simulink model "forcaster"  (Simulink 10.1)
settings: Solver=FixedStepAuto  StartTime=0.0  StopTime=10.0  FixedStep=DT  RelTol=1e-3
values from neighbouring files (symbols this model uses):
  T_s = 0.1    [run_Top_Model.m]
undefined symbols (not defined in the file or in its folder): DiscIntNeverNeededParam, T_mean, T_r
libraries: ctrlSharedLib x2, dspmtrx3 x1
settings Model: Creator=lpwoolcock  LastModifiedBy=arthu
settings DataIOCC: SaveFormat=Dataset  ReturnWorkspaceOutputs=on
settings OptimizationCC: LifeSpan=auto
settings DebuggingCC: UnderspecifiedInitializationDetection=Simplified  MergeDetectMultiDrivingBlocksExec=error  SFUnexpectedBacktrackingDiag=error  SFNoUnconditionalDefaultTransitionDiag=error  SFExecutionAtInitializationDiag=warning  ArithmeticOperatorsInVariantConditions=error
settings HardwareCC: ProdBitPerPointer=64  ProdBitPerSizeT=64  ProdBitPerPtrDiffT=64  ProdLargestAtomicFloat=Float  ProdIntDivRoundTo=Zero  ProdEndianess=LittleEndian  ProdWordSize=64  ProdHWDeviceType=Intel->x86-64 (Windows64)
settings ModelReferenceCC: PropagateSignalLabelsOutOfModel=on
settings SFSimCC: SimUseLocalCustomCode=on  CustomCodeUndefinedFunction=FilterOut
settings RTWCC: RTWUseLocalCustomCode=on
settings CodeAppCC: StateflowObjectComments=off
settings GRTTargetCC: TargetLangStandard=C99 (ISO)  CombineOutputUpdateFcns=on  GRTInterface=off
settings ConfigComp: CovMetricSettings=dwe  CovHtmlReporting=off  CovSaveCumulativeToWorkspaceVar=off  CovSaveSingleToWorkspaceVar=off  CovExternalEMLEnable=on

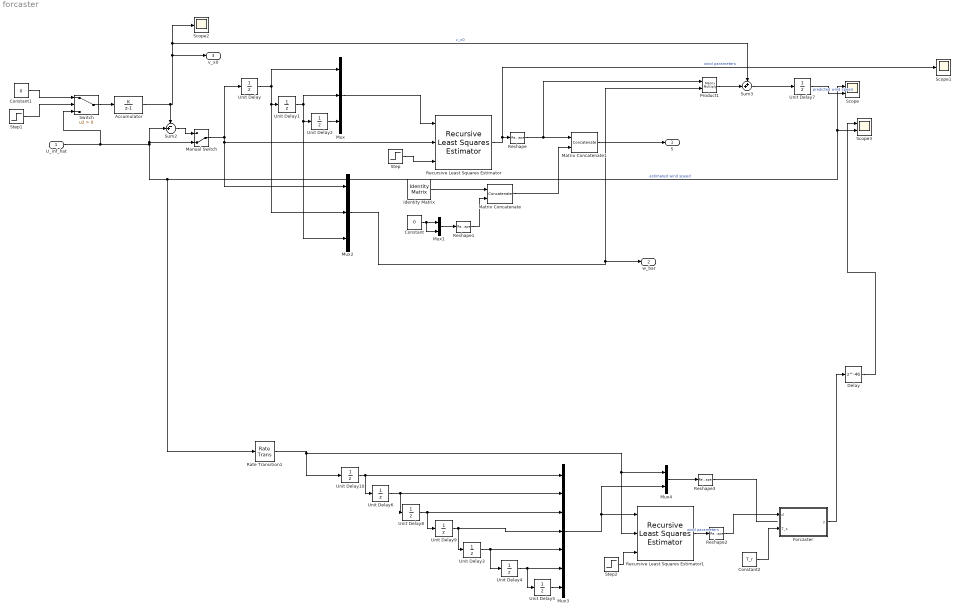
== system forcaster ==
  U_inf_hat : Inport  SampleTime=T_s
  Accumulator : DiscreteIntegrator  IntegratorMethod=Accumulation: Forward Euler  gainval=T_s/T_mean  SampleTime=T_s  ICPrevOutput=DiscIntNeverNeededParam  ICPrevScaledInput=DiscIntNeverNeededParam
  Constant : Constant  Value=0
  Constant1 : Constant  Value=0
  Constant2 : Constant  Value=T_r
  Delay : Delay  DelayLength=46  InitialCondition=0
  Forcaster : MATLAB Function  TreatAsAtomicUnit=on
  Identity Matrix : dspmtrx3/Identity Matrix  Inherit=off  N=2  Ts=T_s  dataType=double  isSigned=on  wordLen=16  udDataType=sfix(16)  fracBitsMode=Best precision  numFracBits=15  OutDataTypeStr=double  LastOutDataTypeStr=double
  Manual Switch : ManualSwitch  CurrentSetting=0
  Matrix Concatenate : Concatenate  Mode=Multidimensional array  ConcatenateDimension=2
  Matrix Concatenate1 : Concatenate  Mode=Multidimensional array
  Mux : Mux  Inputs=3
  Mux1 : Mux  Inputs=2
  Mux2 : Mux  Inputs=3
  Mux3 : Mux  Inputs=7
  Mux4 : Mux  Inputs=2
  Product1 : Product  Multiplication=Matrix(*)
  Rate Transition1 : RateTransition  Deterministic=off  OutPortSampleTime=T_r
  Recursive Least Squares Estimator : ctrlSharedLib/Recursive Least Squares Estimator  InitialEstimateSource=None  InitialParameterData=3  P0=1e4  InitialRegressors=0  InitialOutputs=0  History=Infinite  WindowLength=200  EstimationMethod=Forgetting Factor  AdaptationParameter=0.9  HasTimeVaryingAdaptationParameter=off  NormalizationBias=eps  OutputError=off  OutputP=off  AddEnablePort=off  ExternalReset=Rising  InputProcessing=Sample-based  Ts=-1
      settings: SourceProductBaseCode=CT,ID
  Recursive Least Squares Estimator1 : ctrlSharedLib/Recursive Least Squares Estimator  InitialEstimateSource=None  InitialParameterData=7  P0=1e4  InitialRegressors=0  InitialOutputs=0  History=Infinite  WindowLength=200  EstimationMethod=Forgetting Factor  AdaptationParameter=0.99  HasTimeVaryingAdaptationParameter=off  NormalizationBias=eps  OutputError=off  OutputP=off  AddEnablePort=off  ExternalReset=Rising  InputProcessing=Sample-based  Ts=T_r
      settings: SourceProductBaseCode=CT,ID
  Reshape : Reshape  OutputDimensionality=Row vector (2-D)
  Reshape1 : Reshape  OutputDimensionality=Column vector (2-D)
  Reshape2 : Reshape  OutputDimensionality=Row vector (2-D)
  Reshape3 : Reshape  OutputDimensionality=Column vector (2-D)
  Scope : Scope  NumInputPorts=2
  Scope1 : Scope
  Scope2 : Scope
  Scope3 : Scope  NumInputPorts=2
  Step : Step  Time=T_mean  SampleTime=T_s
  Step1 : Step  Time=T_mean  SampleTime=T_s
  Step2 : Step  Time=T_mean  SampleTime=T_s
  Sum2 : Sum  Inputs=-+|
  Sum3 : Sum  Inputs=++|
  Switch : Switch  Criteria=u2 > Threshold
  Unit Delay{,1..10} (11 alike) : UnitDelay  SampleTime=-1  HasFrameUpgradeWarning=on
  S : Outport  SampleTime=T_s
  w_bar : Outport  Port=2  SampleTime=T_s
  v_x0 : Outport  Port=3  SampleTime=T_s
  wires:
  Matrix Concatenate/1 -> Matrix Concatenate1/2
  Mux/1 -> Recursive Least Squares Estimator/1
  Unit Delay2/1 -> Mux/3
  Matrix Concatenate1/1 -> S/1
  Reshape/1 -> Product1/1, Matrix Concatenate1/1
  Constant/1 -> Mux1/2, Mux1/1
  Reshape1/1 -> Matrix Concatenate/2
  Mux1/1 -> Reshape1/1
  Unit Delay1/1 -> Mux/2, Mux2/3, Unit Delay2/1
  Recursive Least Squares Estimator/1 -> Scope1/1, Reshape/1  "wind parameters"
  Identity Matrix/1 -> Matrix Concatenate/1
  Unit Delay/1 -> Mux/1, Mux2/2, Unit Delay1/1
  Mux2/1 -> w_bar/1, Product1/2
  Unit Delay7/1 -> Scope/2  "predicted wind speed"
  U_inf_hat/1 -> Switch/3, Manual Switch/2, Sum2/2, Rate Transition1/1, Scope/1, Scope3/2  "estimated wind speed"
  Manual Switch/1 -> Mux2/1, Recursive Least Squares Estimator/2, Unit Delay/1
  Sum3/1 -> Unit Delay7/1
  Step/1 -> Recursive Least Squares Estimator/3
  Step1/1 -> Switch/2
  Constant1/1 -> Switch/1
  Switch/1 -> Accumulator/1
  Accumulator/1 -> Sum2/1, v_x0/1, Sum3/1, Scope2/1  "v_x0"
  Product1/1 -> Sum3/2
  Constant2/1 -> Forcaster/2(T_s)
  Sum2/1 -> Manual Switch/1
  Unit Delay5/1 -> Mux3/7
  Unit Delay4/1 -> Unit Delay5/1, Mux3/6
  Unit Delay3/1 -> Unit Delay4/1, Mux3/5
  Unit Delay9/1 -> Unit Delay3/1, Mux3/4
  Unit Delay8/1 -> Unit Delay9/1, Mux3/3
  Unit Delay6/1 -> Unit Delay8/1, Mux3/2
  Unit Delay10/1 -> Unit Delay6/1, Mux3/1
  Step2/1 -> Recursive Least Squares Estimator1/3
  Mux3/1 -> Mux4/2, Recursive Least Squares Estimator1/1
  Recursive Least Squares Estimator1/1 -> Reshape2/1  "wind parameters"
  Reshape2/1 -> Forcaster/1(d)
  Reshape3/1 -> ?
  Mux4/1 -> Reshape3/1
  Rate Transition1/1 -> Mux4/1, Recursive Least Squares Estimator1/2, Unit Delay10/1
  Forcaster/1(y) -> Delay/1
  Delay/1 -> Scope3/1

== matlab function Forcaster ==
  data: d input double; y output double; T_s input double


function y = forcaster_2(d,T_s)

forTime = 4.6;                  %time forcast
num_for = ceil(forTime/T_s);    
order = 100;                    %order of regression
delta = 1;                      %initialisation param
lambda = 0.9;                   %forgetting factor

%set up registers
persistent U;
if(isempty(U))
   U = zeros(order,1);
end

persistent Z;
if(isempty(Z))
   Z = zeros(order,1);
end


persistent P;
if(isempty(P)) 
    P = eye(size(U,1))*delta;
end

%recursive least squares
K = P*U/(lambda+U'*P*U);
zeta = d-Z'*U;
Z = Z+K*zeta;
P = P/lambda-K*U'*P/lambda;

%update register
U(2:end,1) = U(1:end-1,1)
U(1,1) = d; 

S = [Z';eye(order-1) zeros(order-1,1)];
Y = S^num_for*U;
y = Y(1,1)
if(y>30) %saturation
    y = 30;
end
end
